simulink model "ER_level_flight2"  (R2016b)
settings: Solver=ode45  StartTime=0.01  StopTime=50  RelTol=1e-3  EnableMultiTasking=on
undefined symbols (not defined in the file or in its folder): sigbuilder_block
libraries: aerolibtransform2 x1
settings Model: Creator=Administrator  LastModifiedBy=maelula
settings DataIOCC: LimitDataPoints=on  SaveFormat=Array
settings OptimizationCC: LifeSpan=inf
settings DebuggingCC: SolverPrmCheckMsg=warning  SFUnexpectedBacktrackingDiag=warning  SFNoUnconditionalDefaultTransitionDiag=warning  SFExecutionAtInitializationDiag=none
settings HardwareCC: ProdBitPerPointer=32  ProdBitPerSizeT=32  ProdBitPerPtrDiffT=32  ProdLargestAtomicFloat=None  ProdIntDivRoundTo=Undefined  ProdEndianess=Unspecified  ProdWordSize=32  ProdHWDeviceType=32-bit Generic
settings ModelReferenceCC: PropagateSignalLabelsOutOfModel=off
settings GRTTargetCC: TargetLangStandard=C89/C90 (ANSI)
settings ConfigComp: CovMetricSettings=dw  CovSaveCumulativeToWorkspaceVar=on  CovSaveSingleToWorkspaceVar=on  CovExternalEMLEnable=off  CovSFcnEnable=off

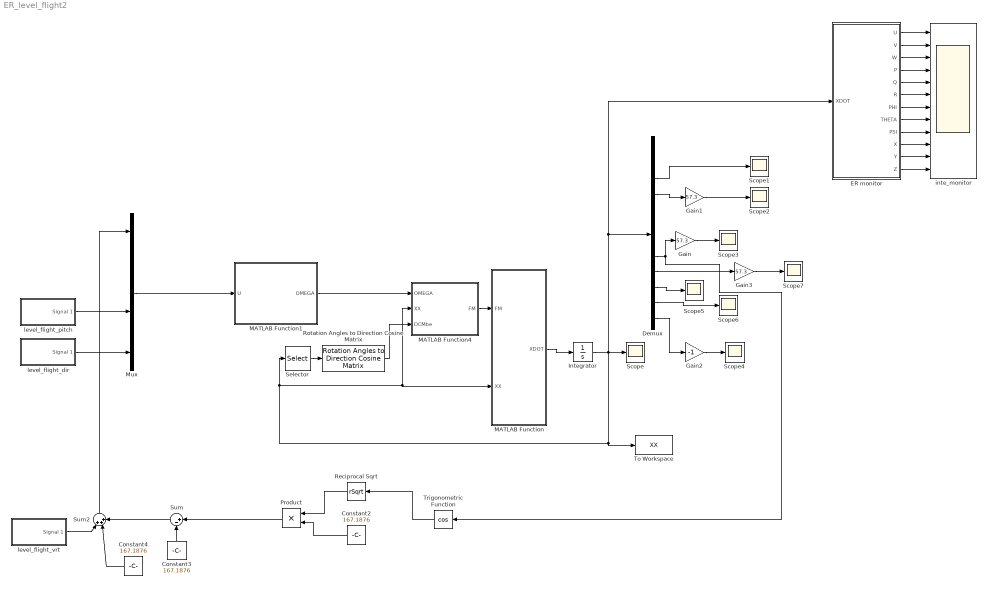
== system ER_level_flight2 ==
  Constant2 : Constant  Value=167.1876
  Constant3 : Constant  Value=167.1876
  Constant4 : Constant  Value=167.1876
  Demux : Demux  Outputs=12
  ER monitor : MATLAB Function  TreatAsAtomicUnit=on
  Gain : Gain  Gain=57.3
  Gain1 : Gain  Gain=57.3
  Gain2 : Gain  Gain=-1
  Gain3 : Gain  Gain=57.3
  Integrator : Integrator
  MATLAB Function : MATLAB Function  TreatAsAtomicUnit=on
  MATLAB Function1 : MATLAB Function  TreatAsAtomicUnit=on
  MATLAB Function4 : MATLAB Function  TreatAsAtomicUnit=on
  Mux : Mux
  Product : Product
  Reciprocal Sqrt : Sqrt  Operator=rSqrt  SaturateOnIntegerOverflow=on
  Rotation Angles to Direction Cosine Matrix : aerolibtransform2/Rotation Angles to Direction Cosine Matrix  rotationOrder=ZYX
  Scope{,1..7} (8 alike) : Scope
  Selector : Selector  InputPortWidth=12  IndexOptions=Index vector (dialog)  Indices=[9 8 7]  OutputSizes=1
  Sum : Sum  Inputs=|+-
  Sum2 : Sum  Inputs=|+++
  To Workspace : ToWorkspace  VariableName=XX  SampleTime=-1
  Trigonometric Function : Trigonometry  Operator=cos
  inte_monitor : Scope  NumInputPorts=12
  level_flight_dir : Subsystem  Tag=STV Subsys  LoadFcn=sigbuilder_block('load');  StartFcn=sigbuilder_block('start');  StopFcn=sigbuilder_block('stop');  ClipboardFcn=sigbuilder_block('clipboard');  mask(Sigbuilder block){tuvar=[0:10]}
      mask help: Simulink:masks:SigbuilderBlock_MD
      mask init:
      | if ~strcmp(get_param(bdroot(gcbh),'SimulationStatus'),'stopped') tuvar = sigbuilder_block('maskInit'); end
      settings: CopyFcn=sigbuilder_block('copy');  DeleteFcn=sigbuilder_block('delete');  ModelCloseFcn=sigbuilder_block('modelClose');  PreSaveFcn=sigbuilder_block('preSave');  PauseFcn=sigbuilder_block('pause');  ContinueFcn=sigbuilder_block('continue');  NameChangeFcn=sigbuilder_block('namechange');  OpenFcn=sigbuilder_block('open',[288 188 781 555 ]);  CloseFcn=sigbuilder_block('close');
      mask Display: plot(0, 0, 100, 100,[2, 2, 32, 32, 2], [68, 8, 8, 68, 68],[32, 2], [38, 38], [32, 19, 2],[53, 60, 44], [32, 17, 17, 2],[16, 16, 31, 31]);txt = getActiveGroup(gcbh);text(2, 100, txt,'verticalAlignment', 'top');
  level_flight_pitch : Subsystem  Tag=STV Subsys  LoadFcn=sigbuilder_block('load');  StartFcn=sigbuilder_block('start');  StopFcn=sigbuilder_block('stop');  ClipboardFcn=sigbuilder_block('clipboard');  mask(Sigbuilder block){tuvar=[0:10]}
      mask help: Simulink:masks:SigbuilderBlock_MD
      mask init:
      | if ~strcmp(get_param(bdroot(gcbh),'SimulationStatus'),'stopped') tuvar = sigbuilder_block('maskInit'); end
      settings: CopyFcn=sigbuilder_block('copy');  DeleteFcn=sigbuilder_block('delete');  ModelCloseFcn=sigbuilder_block('modelClose');  PreSaveFcn=sigbuilder_block('preSave');  PauseFcn=sigbuilder_block('pause');  ContinueFcn=sigbuilder_block('continue');  NameChangeFcn=sigbuilder_block('namechange');  OpenFcn=sigbuilder_block('open',[301 190 826 540 ]);  CloseFcn=sigbuilder_block('close');
      mask Display: plot(0, 0, 100, 100,[2, 2, 32, 32, 2], [68, 8, 8, 68, 68],[32, 2], [38, 38], [32, 19, 2],[53, 60, 44], [32, 17, 17, 2],[16, 16, 31, 31]);txt = getActiveGroup(gcbh);text(2, 100, txt,'verticalAlignment', 'top');
  level_flight_vrt : Subsystem  Tag=STV Subsys  LoadFcn=sigbuilder_block('load');  StartFcn=sigbuilder_block('start');  StopFcn=sigbuilder_block('stop');  ClipboardFcn=sigbuilder_block('clipboard');  mask(Sigbuilder block){tuvar=[0:10]}
      mask help: Simulink:masks:SigbuilderBlock_MD
      mask init:
      | if ~strcmp(get_param(bdroot(gcbh),'SimulationStatus'),'stopped') tuvar = sigbuilder_block('maskInit'); end
      settings: CopyFcn=sigbuilder_block('copy');  DeleteFcn=sigbuilder_block('delete');  ModelCloseFcn=sigbuilder_block('modelClose');  PreSaveFcn=sigbuilder_block('preSave');  PauseFcn=sigbuilder_block('pause');  ContinueFcn=sigbuilder_block('continue');  NameChangeFcn=sigbuilder_block('namechange');  OpenFcn=sigbuilder_block('open',[255 190 838 517 ]);  CloseFcn=sigbuilder_block('close');
      mask Display: plot(0, 0, 100, 100,[2, 2, 32, 32, 2], [68, 8, 8, 68, 68],[32, 2], [38, 38], [32, 19, 2],[53, 60, 44], [32, 17, 17, 2],[16, 16, 31, 31]);txt = getActiveGroup(gcbh);text(2, 100, txt,'verticalAlignment', 'top');
  wires:
  MATLAB Function1/1(OMEGA) -> MATLAB Function4/1(OMEGA)
  Mux/1 -> MATLAB Function1/1(U)
  MATLAB Function4/1(FM) -> MATLAB Function/1(FM)
  MATLAB Function/1(XDOT) -> Integrator/1
  Selector/1 -> Rotation Angles to Direction Cosine Matrix/1
  Rotation Angles to Direction Cosine Matrix/1 -> MATLAB Function4/3(DCMbe)
  Demux/3 -> Scope1/1
  Demux/10 -> Scope5/1
  Demux/11 -> Scope6/1
  Demux/4 -> Gain1/1
  Gain1/1 -> Scope2/1
  Demux/8 -> Trigonometric Function/1, Gain/1
  Demux/12 -> Gain2/1
  Gain2/1 -> Scope4/1
  level_flight_dir/1(Signal 1) -> Mux/4
  Demux/9 -> Gain3/1
  Gain3/1 -> Scope7/1
  Gain/1 -> Scope3/1
  Trigonometric Function/1 -> Reciprocal Sqrt/1
  Reciprocal Sqrt/1 -> Product/1
  Constant2/1 -> Product/2
  Product/1 -> Sum/1
  Constant3/1 -> Sum/2
  Sum2/1 -> Mux/1
  level_flight_pitch/1(Signal 1) -> Mux/3
  Constant4/1 -> Sum2/2
  ER monitor/2(V) -> inte_monitor/2
  ER monitor/4(P) -> inte_monitor/4
  ER monitor/5(Q) -> inte_monitor/5
  ER monitor/6(R) -> inte_monitor/6
  ER monitor/8(THETA) -> inte_monitor/8
  ER monitor/11(Y) -> inte_monitor/11
  ER monitor/7(PHI) -> inte_monitor/7
  ER monitor/9(PSI) -> inte_monitor/9
  ER monitor/10(X) -> inte_monitor/10
  Integrator/1 -> To Workspace/1, Selector/1, MATLAB Function/2(XX), MATLAB Function4/2(XX), ER monitor/1(XDOT), Demux/1, Scope/1
  ER monitor/12(Z) -> inte_monitor/12
  ER monitor/3(W) -> inte_monitor/3
  ER monitor/1(U) -> inte_monitor/1
  level_flight_vrt/1(Signal 1) -> Sum2/1
  Sum/1 -> Sum2/3

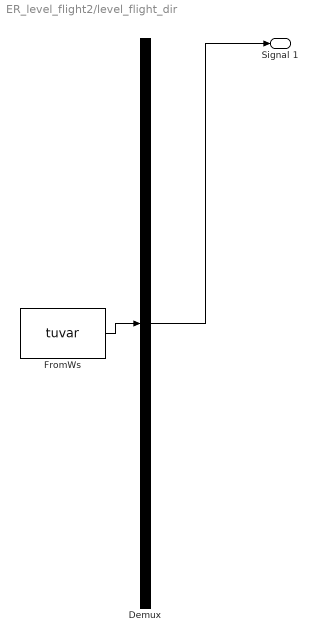
== system ER_level_flight2/level_flight_dir ==
  Demux : Demux  Tag=STV Demux  Outputs=1
  FromWs : FromWorkspace  Tag=STV FromWs  VariableName=tuvar  SampleTime=0
      SigBuilderData=|
      | common.afterFinalStr = 'Extrapolate'
      | common.sampleTime = 0
      | dataSet.timeRange = [0 10]
      | dataSet.name = 'Group 1'
      | sbobj.Groups.Name = 'Group 1'
      | sbobj.Groups.Signals.Name = 'Signal 1'
      | sbobj.Groups.Signals.XData = [0 4 4 4.4 4.4 10]
      | sbobj.Groups.Signals.YData = [0 0 177.97 177.97 0 0]
  Signal 1 : Outport  Tag=STV Outport
  wires:
  Demux/1 -> Signal 1/1
  FromWs/1 -> Demux/1

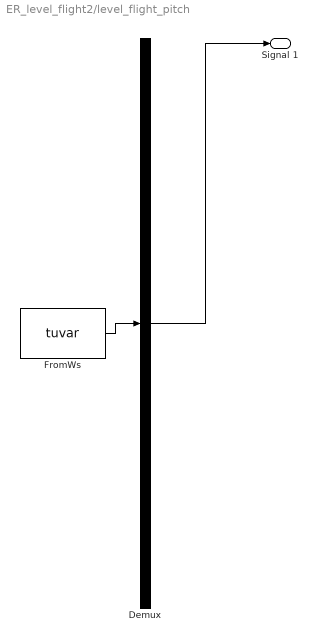
== system ER_level_flight2/level_flight_pitch ==
  Demux : Demux  Tag=STV Demux  Outputs=1
  FromWs : FromWorkspace  Tag=STV FromWs  VariableName=tuvar  SampleTime=0
      SigBuilderData=|
      | common.afterFinalStr = 'Extrapolate'
      | common.sampleTime = 0
      | dataSet.timeRange = [0 10]
      | dataSet.name = 'Group 1'
      | sbobj.Groups.Name = 'Group 1'
      | sbobj.Groups.Signals.Name = 'Signal 1'
      | sbobj.Groups.Signals.XData = [0 4.5 4.5 4.9 4.9 10]
      | sbobj.Groups.Signals.YData = [0 0 62.895 62.895 0 0]
  Signal 1 : Outport  Tag=STV Outport
  wires:
  Demux/1 -> Signal 1/1
  FromWs/1 -> Demux/1

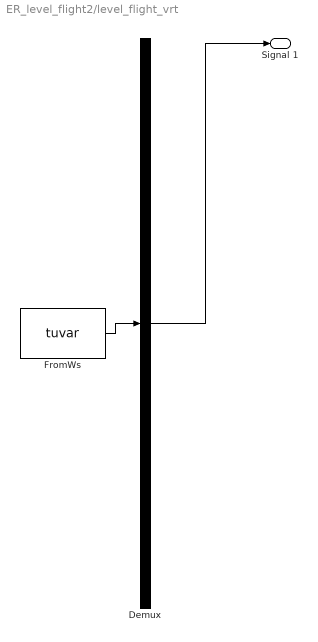
== system ER_level_flight2/level_flight_vrt ==
  Demux : Demux  Tag=STV Demux  Outputs=1
  FromWs : FromWorkspace  Tag=STV FromWs  VariableName=tuvar  SampleTime=0
      SigBuilderData=|
      | common.afterFinalStr = 'Extrapolate'
      | common.sampleTime = 0
      | dataSet.timeRange = [0 10]
      | dataSet.name = 'Group 1'
      | sbobj.Groups.Name = 'Group 1'
      | sbobj.Groups.Signals.Name = 'Signal 1'
      | sbobj.Groups.Signals.XData = [0 1 1 4 10]
      | sbobj.Groups.Signals.YData = [32.8124 32.8124 32.8124 0 0]
  Signal 1 : Outport  Tag=STV Outport
  wires:
  Demux/1 -> Signal 1/1
  FromWs/1 -> Demux/1

== matlab function ER_level_flight2/MATLAB Function1 ==
  data: U input; OMEGA output
function OMEGA  =change(U)

Rvrt = U(1);
Rroll = U(2);
Rpitch = U(3);
Rdir = U(4);

a1=Rvrt*Rvrt;
a2=Rroll*Rroll;
a3=Rpitch*Rpitch;
a4=Rdir*Rdir;

R1=a1+a2+a3-a4;
R2=a1-a2+a3+a4;
R3=a1-a2-a3-a4;
R4=a1+a2-a3+a4;
R5=a1+a2+a3+a4;
R6=a1-a2+a3-a4;
R7=a1-a2-a3+a4;
R8=a1+a2-a3-a4;
%
OMEGA = [R1;R2;R3;R4;R5;R6;R7;R8];

== matlab function ER_level_flight2/MATLAB Function ==
  data: FM input; XX input; XDOT output
function XDOT =dynamics(FM,XX)
%
U = XX(1,1);
V = XX(2,1);
W = XX(3,1);
P = XX(4,1);
Q = XX(5,1);
R = XX(6,1);
PHI = XX(7,1);
THETA = XX(8,1);
PSI = XX(9,1);
X = XX(10,1);
Y = XX(11,1);
Z = XX(12,1);

FX = FM(1);
FY = FM(2);
FZ = FM(3);
MX = FM(4);
MY = FM(5);
MZ = FM(6);


m = 1.6;
g = 9.81;

IX = 0.0081;
IY = 0.0081;
IZ = 0.00142;

IZX = 0;

L = MX;
M = MY;
N = MZ;


Ut = V*R-W*Q+FX/m;
Vt = -U*R+W*P+FY/m;
Wt = U*Q-V*P+FZ/m;

Pt = 1/(IX*IZ-IZX^2)*(IZ*L+IZX*N+IZX*(IX-IY+IZ)*P*Q+(IY*IZ-IZX^2-IZ^2)*Q*R);
Qt = 1/(IY)*(M-(IX-IZ)*P*R-IZX*(P^2-R^2));
Rt = 1/(IX*IZ-IZX^2)*(IZX*L+IX*N+(IX^2-IX*IY+IZX^2)*P*Q-IZX*(IX-IY-IZ)*Q*R);

PHIt = P+tan(THETA)*(Q*sin(PHI)+R*cos(PHI));
THETAt = Q*cos(PHI)-R*sin(PHI);
PSIt = 1/cos(PHI)*(Q*sin(PHI)+R*cos(PHI));

Xt = U*cos(THETA)*cos(PSI)+V*(sin(THETA)*sin(PHI)*cos(PSI)-cos(PHI)*sin(PSI))+W*(sin(THETA)*cos(PHI)*cos(PSI)+sin(PHI)*sin(PSI));
Yt = U*cos(THETA)*sin(PSI)+V*(sin(THETA)*sin(PHI)*sin(PSI)+cos(PHI)*cos(PSI))+W*(sin(THETA)*cos(PHI)*sin(PSI)-sin(PHI)*cos(PSI));
Zt = -U*sin(THETA)+V*sin(PHI)*cos(THETA)+W*cos(PHI)*cos(THETA);

XDOT = [Ut,Vt,Wt,Pt,Qt,Rt,PHIt,THETAt,PSIt,Xt,Yt,Zt]';

== matlab function ER_level_flight2/ER monitor ==
  data: XDOT input; U output; V output; W output; P output; Q output; R output; PHI output; THETA output; PSI output; X output; Y output; Z output
function [U,V,W,P,Q,R,PHI,THETA,PSI,X,Y,Z] = monitor(XDOT)

% y1 = XDOT(1);
% y2 = XDOT(1);
% y3 = XDOT(1);
% y4 = XDOT(1);
% y5 = XDOT(1);
% y6 = XDOT(1);
% y7 = XDOT(1);
% y8 = XDOT(1);
% y9 = XDOT(1);
% y10 = XDOT(1);
% y11 = XDOT(1);
% y12 = XDOT(1);

U = -XDOT(1);
V = -XDOT(2);
W = -XDOT(3);
P = XDOT(4);
Q = XDOT(5);
R = XDOT(6);
PHI = XDOT(7);
THETA = XDOT(8);
PSI = XDOT(9);
X = -XDOT(10);
Y = -XDOT(11);
Z = -XDOT(12);

== matlab function ER_level_flight2/MATLAB Function4 ==
  data: OMEGA input; FM output; XX input; DCMbe input
function FM= MATLAB_Function4(OMEGA, XX, DCMbe)
%旋翼力%
Fx1=0;
Fy1=0;
l=0.5;
ll=sqrt(2);
rou=1.225;
k1=5.73*10^(-5);
k2=2.53*10^(-6);

OMEGA1S=OMEGA(1);
OMEGA2S=OMEGA(2);
OMEGA3S=OMEGA(3);
OMEGA4S=OMEGA(4);
OMEGA5S=OMEGA(5);
OMEGA6S=OMEGA(6);
OMEGA7S=OMEGA(7);
OMEGA8S=OMEGA(8);

L1=rou*k1*OMEGA1S;
L2=rou*k1*OMEGA2S;
L3=rou*k1*OMEGA3S;
L4=rou*k1*OMEGA4S;
L5=rou*k1*OMEGA5S;
L6=rou*k1*OMEGA6S;
L7=rou*k1*OMEGA7S;
L8=rou*k1*OMEGA8S;

Fz1=-(L1+L2+L3+L4+L5+L6+L7+L8);
Mx1=1/ll*l*(L1-L2-L3+L4+L5-L6-L7+L8);
My1=1/ll*l*(L1+L2-L3-L4+L5+L6-L7-L8);
Mz1=k2/k1*(-L1+L2-L3+L4+L5-L6+L7-L8);
%气动力
CD=0.8;
u=XX(1,1);
v=XX(2,1);
w=XX(3,1);
V=(u^2+v^2+w^2)^0.5;

p=XX(4,1);
q=XX(5,1);
r=XX(6,1);



Ax=-CD*V*u;
Ay=-CD*V*v;
Az=-CD*V*w;

AMx=-CD*0.5*p;
AMy=-CD*0.5*q;
AMz=-CD*0.5*r;
%重力
m = 1.6;
g = 9.81;
gforce = DCMbe*[0,0,m*g]';
Fx=Fx1+Ax+gforce(1);
Fy=Fy1+Ay+gforce(2);
Fz=Fz1+Az+gforce(3);
Mx=Mx1+AMx;
My=My1+AMy;
Mz=Mz1+AMz;
FM=[Fx,Fy,Fz,Mx,My,Mz]';
